simulink model "test_pkt_reorder"  (Simulink 6.2)
settings: Solver=ode45  StartTime=0.0  StopTime=200000  RelTol=1e-3
libraries: xbsIndex_r3 x556, casper_library x22, xps_library x21, simulink x1
(part 1 of 3)
settings Model: LastModifiedBy=dsp
settings DebuggingCC: SolverPrmCheckMsg=warning

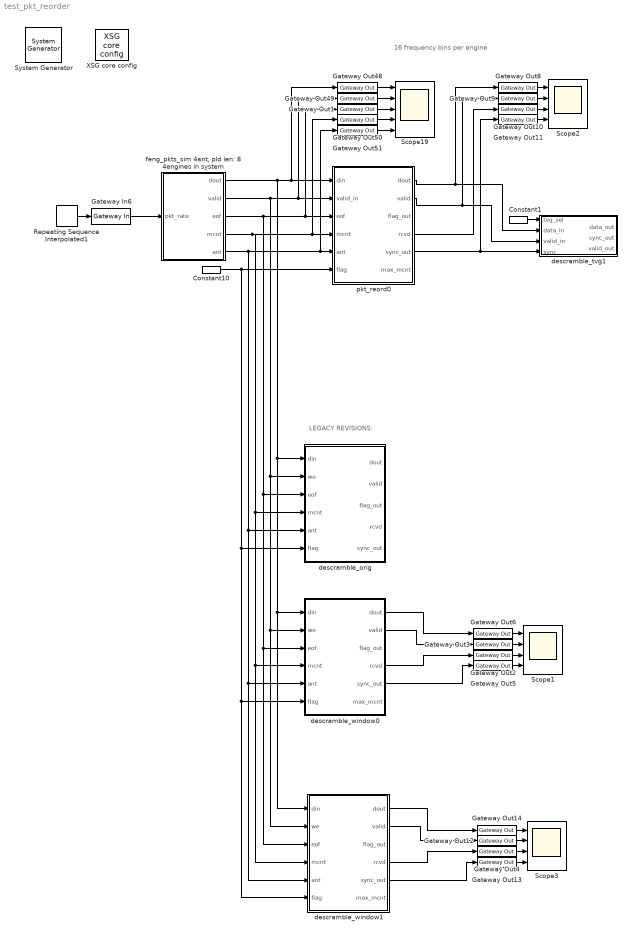
== system test_pkt_reorder ==
  note: 16 frequency bins per engine
  note: LEGACY REVISIONS:
  " System Generator" : xbsIndex_r3/ System Generator  Tag=genX  xilinxfamily=Virtex2  part=xc2v1000  speed=-4  package=bg575  synthesis_tool=XST  directory=./netlist  testbench=off  simulink_period=1  sysclk_period=100  incr_netlist=off  trim_vbits=Everywhere in SubSystem  dbl_ovrd=According to Block Masks  core_generation=According to Block Masks  run_coregen=off  deprecated_control=off  eval_field=0
      settings: AttributesFormatString=System\nGenerator
  Constant1 : xbsIndex_r3/Constant  const=0  equ=P=C  arith_type=Unsigned  n_bits=2  bin_pt=0  opselect=C  inp2=PCIN>>17  opr=+  inp1=P  carry=CIN  iostate=0  explicit_period=on  period=1  dbl_ovrd=off
  Constant10 : xbsIndex_r3/Constant  const=0  equ=P=C  arith_type=Unsigned  n_bits=1  bin_pt=0  opselect=C  inp2=PCIN>>17  opr=+  inp1=P  carry=CIN  iostate=0  explicit_period=on  period=1  dbl_ovrd=off
  Gateway In6 : xbsIndex_r3/Gateway In  arith_type=Unsigned  n_bits=1  bin_pt=0  quantization=Truncate  overflow=Wrap  period=1  timing_constraint=None  locs_specified=off  LOCs={}  needs_fixed_name=off  dbl_ovrd=off  show_param=off
      settings: xl_area=[0, 0, 0, 0, 0, 0, 0]
  Gateway Out{1..6,8..14,48..51} (17 alike) : xbsIndex_r3/Gateway Out  output_type=Double  nbits=8  bin_pt=6  arith_type=Boolean  quantization=Truncate  overflow=Wrap  hdl_port=on  timing_constraint=None  locs_specified=off  LOCs={}  needs_fixed_name=off  show_param=off
      settings: xl_area=[0, 0, 0, 0, 0, 0, 0]
  Repeating Sequence Interpolated1 : simulink/Sources/Repeating Sequence Interpolated  OutValues=[0 1].'  TimeValues=[50000 100000].'  LookUpMeth=Use Input Above  tsamp=1  OutputDataTypeScalingMode=Specify via dialog  OutDataType=float('double')  OutScaling=2^-10
  Scope1 : Scope  NumInputPorts=4
      settings: YMin=0~0~0~-1  YMax=1~1~1~1  SaveName=ScopeData5
  Scope19 : Scope  NumInputPorts=5
      settings: YMin=0~0~0~0~0  YMax=3e+014~1~1~3000~3  SaveName=ScopeData2
  Scope2 : Scope  NumInputPorts=4
      settings: YMin=0~0~0~-1  YMax=1~1~1~1
  Scope3 : Scope  NumInputPorts=4
      settings: YMin=0~0~0~-1  YMax=1~1~1~1  SaveName=ScopeData6
  XSG core config : xps_library/XSG core config  Tag=xps:xsg  hw_sys=BEE2_usr  ibob_linux=off  clk_src=sys_clk  gpio_clk_io_group=iBOB:sma  gpio_clk_bit_index=0  clk_rate=205  sample_period=1  synthesis_tool=XST  mpc_type=powerpc405
  descramble_orig : Subsystem  mask{ant_bits=2, x_int_bits=5, window_bits=3, sync_bits=11}
      mask prompts: ant_bits "Maximum Number of Antennas (2^?):"; x_int_bits "X Engine Integration Length (2^?):"; window_bits "Number of Windows to Buffer (2^?):"; sync_bits "Samples Between Sync Pulses (2^?)"
  descramble_tvg1 : Subsystem  mask{ant_bits=2, x_int_bits=5, sync_period=15}
      mask prompts: ant_bits "Number of Antennas (2^?):"; x_int_bits "X Integration Length (2^?):"; sync_period "Sync Pulse Period (2^?):"
  descramble_window0 : Subsystem  mask{ant_bits=2, xeng_bits=2, chan_bits=6, x_int_bits=5, window_bits=3}
      mask prompts: ant_bits "Maximum Number of Antennas (2^?):"; xeng_bits "Number of Xengines in the system (2^?)"; chan_bits "Number of frequency channels in the system (2^?)"; x_int_bits "X Engine Integration Length (2^?):"; window_bits "Number of Windows to Buffer (2^?):"
      mask init:
      | sync_bits=chan_bits+x_int_bits+ant_bits-xeng_bits
      | 
      | fmtstr = sprintf('Sync period: 2^%d\nPayload Len: %i', sync_bits,2^(x_int_bits - 2));
      | set_param(gcb, 'AttributesFormatString', fmtstr);
      settings: AttributesFormatString=|
      | Sync period: 2^11
      | Payload Len: 8
  descramble_window1 : Subsystem  mask{ant_bits=2, xeng_bits=2, chan_bits=6, x_int_bits=5, window_bits=3}
      mask prompts: ant_bits "Maximum Number of Antennas (2^?):"; xeng_bits "Number of Xengines in the system (2^?)"; chan_bits "Number of frequency channels in the system (2^?)"; x_int_bits "X Engine Integration Length (2^?):"; window_bits "Number of Windows to Buffer (2^?):"
      mask init:
      | sync_bits=chan_bits+x_int_bits+ant_bits-xeng_bits
      | 
      | fmtstr = sprintf('Sync period: 2^%d\nPayload Len: %i', sync_bits,2^(x_int_bits - 2));
      | set_param(gcb, 'AttributesFormatString', fmtstr);
      settings: AttributesFormatString=|
      | Sync period: 2^11
      | Payload Len: 8
  "feng_pkts_sim 4ant, pld len: 8 4engines in system" : Subsystem
  pkt_reord0 : Subsystem  mask{ant_bits=3, xeng_bits=3, chan_bits=11, x_int_bits=7, window_bits=3}
      mask prompts: ant_bits "Maximum Number of Antennas (2^?):"; xeng_bits "Number of Xengines in the system (2^?)"; chan_bits "Number of frequency channels in the system (2^?)"; x_int_bits "X Engine Integration Length (2^?):"; window_bits "Number of Windows to Buffer (2^?):"
      mask init:
      | sync_bits=chan_bits+x_int_bits+ant_bits-xeng_bits
      | 
      | fmtstr = sprintf('Sync period: 2^%d\nPayload Len: %i', sync_bits,2^(x_int_bits - 2));
      | set_param(gcb, 'AttributesFormatString', fmtstr);
      settings: AttributesFormatString=|
      | Sync period: 2^18
      | Payload Len: 32
  wires:
  Constant1/1 -> descramble_tvg1/1(tvg_sel)
  Gateway Out8/1 -> Scope2/1
  Gateway Out9/1 -> Scope2/2
  Gateway Out10/1 -> Scope2/3
  Gateway Out11/1 -> Scope2/4
  pkt_reord0/1(dout) -> Gateway Out8/1, descramble_tvg1/2(data_in)
  pkt_reord0/2(valid) -> Gateway Out9/1, descramble_tvg1/3(valid_in)
  pkt_reord0/5(sync_out) -> Gateway Out11/1, descramble_tvg1/4(sync)
  Constant10/1 -> descramble_window0/6(flag), descramble_window1/6(flag), descramble_orig/6(flag), pkt_reord0/6(flag)
  Gateway Out48/1 -> Scope19/1
  Gateway Out49/1 -> Scope19/2
  "feng_pkts_sim 4ant, pld len: 8 4engines in system"/4(mcnt) -> Gateway Out50/1, pkt_reord0/4(mcnt), descramble_window0/4(mcnt), descramble_window1/4(mcnt), descramble_orig/4(mcnt)
  "feng_pkts_sim 4ant, pld len: 8 4engines in system"/1(dout) -> Gateway Out48/1, pkt_reord0/1(din), descramble_window0/1(din), descramble_window1/1(din), descramble_orig/1(din)
  Repeating Sequence Interpolated1/1 -> Gateway In6/1
  "feng_pkts_sim 4ant, pld len: 8 4engines in system"/2(valid) -> Gateway Out49/1, pkt_reord0/2(valid_in), descramble_window0/2(we), descramble_window1/2(we), descramble_orig/2(we)
  Gateway In6/1 -> "feng_pkts_sim 4ant, pld len: 8 4engines in system"/1(pkt_rate)
  "feng_pkts_sim 4ant, pld len: 8 4engines in system"/3(eof) -> Gateway Out1/1, pkt_reord0/3(eof), descramble_window0/3(eof), descramble_window1/3(eof), descramble_orig/3(eof)
  "feng_pkts_sim 4ant, pld len: 8 4engines in system"/5(ant) -> Gateway Out51/1, pkt_reord0/5(ant), descramble_window0/5(ant), descramble_window1/5(ant), descramble_orig/5(ant)
  pkt_reord0/4(rcvd) -> Gateway Out10/1
  Gateway Out50/1 -> Scope19/4
  Gateway Out51/1 -> Scope19/5
  Gateway Out1/1 -> Scope19/3
  Gateway Out6/1 -> Scope1/1
  Gateway Out3/1 -> Scope1/2
  Gateway Out2/1 -> Scope1/3
  Gateway Out5/1 -> Scope1/4
  descramble_window0/1(dout) -> Gateway Out6/1
  descramble_window0/2(valid) -> Gateway Out3/1
  descramble_window0/4(rcvd) -> Gateway Out2/1
  descramble_window0/5(sync_out) -> Gateway Out5/1
  Gateway Out14/1 -> Scope3/1
  Gateway Out12/1 -> Scope3/2
  Gateway Out4/1 -> Scope3/3
  Gateway Out13/1 -> Scope3/4
  descramble_window1/1(dout) -> Gateway Out14/1
  descramble_window1/2(valid) -> Gateway Out12/1
  descramble_window1/4(rcvd) -> Gateway Out4/1
  descramble_window1/5(sync_out) -> Gateway Out13/1

== system test_pkt_reorder/descramble_orig ==
  note: BRAM depth is
      | X int length * # antennas * # windows
  din : Inport  Port=1  LatchInput=off
  we : Inport  Port=2  LatchInput=off
  eof : Inport  Port=3  LatchInput=off
  mcnt : Inport  Port=4  LatchInput=off
  ant : Inport  Port=5  LatchInput=off
  flag : Inport  Port=6  LatchInput=off
  Constant : xbsIndex_r3/Constant  const=0  equ=P=C  arith_type=Unsigned  n_bits=18  bin_pt=0  opselect=C  inp2=PCIN>>17  opr=+  inp1=P  carry=CIN  iostate=0  explicit_period=on  period=1  dbl_ovrd=off
  Constant1 : xbsIndex_r3/Constant  const=0  equ=P=C  arith_type=Unsigned  n_bits=1  bin_pt=0  opselect=C  inp2=PCIN>>17  opr=+  inp1=P  carry=CIN  iostate=0  explicit_period=off  period=1  dbl_ovrd=off
  Delay1 : xbsIndex_r3/Delay  latency=2  reg_retiming=off  explicit_period=off  period=1  en=off  accept_only_valid=off  init_zero=on  dbl_ovrd=off  show_param=off
      settings: xl_area=[0, 0, 0, 0, 0, 0, 0]
  Delay2 : xbsIndex_r3/Delay  latency=4  reg_retiming=off  explicit_period=off  period=1  en=off  accept_only_valid=off  init_zero=on  dbl_ovrd=off  show_param=off
      settings: xl_area=[0, 0, 0, 0, 0, 0, 0]
  Delay3 : xbsIndex_r3/Delay  latency=2  reg_retiming=off  explicit_period=off  period=1  en=off  accept_only_valid=off  init_zero=on  dbl_ovrd=off  show_param=off
      settings: xl_area=[0, 0, 0, 0, 0, 0, 0]
  Delay4 : xbsIndex_r3/Delay  latency=4  reg_retiming=off  explicit_period=off  period=1  en=off  accept_only_valid=off  init_zero=on  dbl_ovrd=off  show_param=off
      settings: xl_area=[0, 0, 0, 0, 0, 0, 0]
  Dual Port RAM : xbsIndex_r3/Dual Port RAM  depth=2^x_int_bits * 2^ant_bits * 2^window_bits  initVector=0  write_mode_A=Read Before Write  write_mode_B=Read Before Write  latency=2  mem_collision=on  init_zero=on  explicit_period=off  period=1  dbl_ovrd=off  rst_a=off  init_a=0  rst_b=off  init_b=0  show_param=off  distributed_mem=off  use_rpm=off  gen_core=off
      settings: xl_area=[0, 0, 0, 0, 0, 0, 0]
  Mux : xbsIndex_r3/Mux  inputs=2  precision=Full  arith_type="Signed  (2's comp)"  n_bits=8  bin_pt=2  quantization=Truncate  overflow=Wrap  latency=0  explicit_period=off  period=1  en=off  dbl_ovrd=off  show_param=off  mux_type=off  use_rpm=off  gen_core=off
      settings: xl_area=[0, 0, 0, 0, 0, 0, 0]
  deflagger : Subsystem
  flagger : Subsystem
  window_addr_gen : Subsystem
  dout : Outport
  valid : Outport  Port=2
  flag_out : Outport  Port=3
  rcvd : Outport  Port=4
  sync_out : Outport  Port=5
  wires:
  window_addr_gen/4(we) -> Dual Port RAM/6
  window_addr_gen/3(wr_addr) -> Dual Port RAM/4
  window_addr_gen/2(re) -> Dual Port RAM/3, Delay1/1
  window_addr_gen/1(rd_addr) -> Dual Port RAM/1
  flagger/1(dout) -> Dual Port RAM/5
  Constant/1 -> Dual Port RAM/2
  deflagger/3(rcvd) -> rcvd/1
  deflagger/2(flag) -> flag_out/1
  deflagger/1(dout) -> dout/1
  Delay1/1 -> valid/1
  we/1 -> window_addr_gen/4(valid)
  eof/1 -> window_addr_gen/3(eof)
  ant/1 -> window_addr_gen/2(ant)
  mcnt/1 -> window_addr_gen/1(mcnt)
  Delay3/1 -> sync_out/1
  window_addr_gen/5(sync_out) -> Delay3/1
  flag/1 -> Delay4/1
  Delay4/1 -> flagger/1(flag)
  din/1 -> Delay2/1
  Delay2/1 -> flagger/2(din)
  Mux/1 -> deflagger/1(din)
  Constant1/1 -> Mux/2
  Dual Port RAM/2 -> Mux/1
  Dual Port RAM/1 -> Mux/3

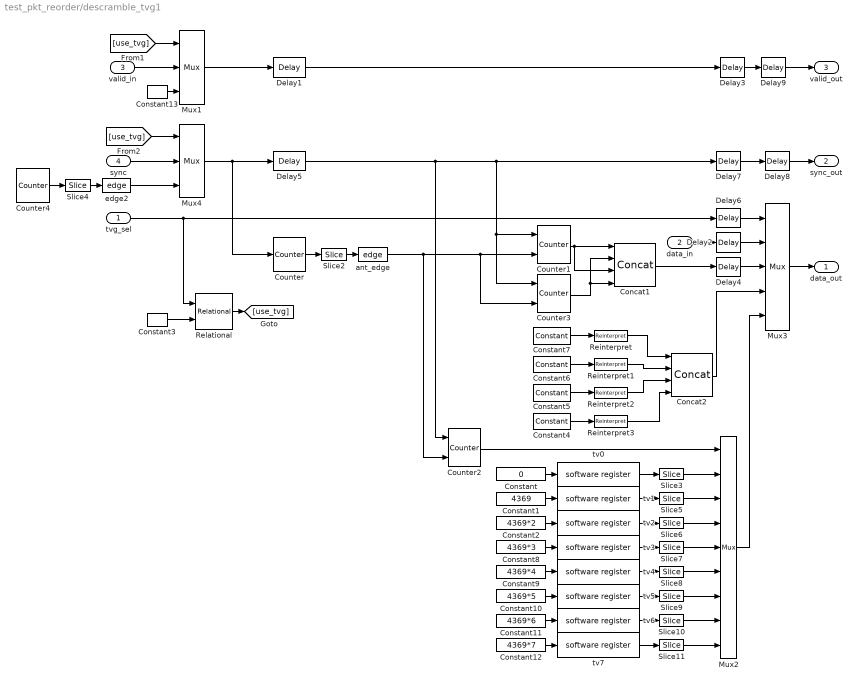
== system test_pkt_reorder/descramble_tvg1 ==
  tvg_sel : Inport  Port=1  LatchInput=off
  data_in : Inport  Port=2  LatchInput=off
  valid_in : Inport  Port=3  LatchInput=off
  sync : Inport  Port=4  LatchInput=off
  Concat1 : xbsIndex_r3/Concat  num_inputs=4  explicit_period=off  period=1  dbl_ovrd=off
  Concat2 : xbsIndex_r3/Concat  num_inputs=4  explicit_period=off  period=1  dbl_ovrd=off
  Constant : Constant  Value=0
  Constant1 : Constant  Value=4369
  Constant10 : Constant  Value=4369*5
  Constant11 : Constant  Value=4369*6
  Constant12 : Constant  Value=4369*7
  Constant13 : xbsIndex_r3/Constant  const=1  equ=P=C  arith_type=Boolean  n_bits=1  bin_pt=0  opselect=C  inp2=PCIN>>17  opr=+  inp1=P  carry=CIN  iostate=0  explicit_period=on  period=1  dbl_ovrd=off
  Constant2 : Constant  Value=4369*2
  Constant3 : xbsIndex_r3/Constant  const=0  equ=P=C  arith_type=Unsigned  n_bits=2  bin_pt=0  opselect=C  inp2=PCIN>>17  opr=+  inp1=P  carry=CIN  iostate=0  explicit_period=on  period=1  dbl_ovrd=off
  Constant4 : xbsIndex_r3/Constant  const=-0.25  equ=P=C  arith_type="Signed  (2's comp)"  n_bits=4  bin_pt=3  opselect=C  inp2=PCIN>>17  opr=+  inp1=P  carry=CIN  iostate=0  explicit_period=on  period=1  dbl_ovrd=off
  Constant5 : xbsIndex_r3/Constant  const=0.5  equ=P=C  arith_type="Signed  (2's comp)"  n_bits=4  bin_pt=3  opselect=C  inp2=PCIN>>17  opr=+  inp1=P  carry=CIN  iostate=0  explicit_period=on  period=1  dbl_ovrd=off
  Constant6 : xbsIndex_r3/Constant  const=-6/8  equ=P=C  arith_type="Signed  (2's comp)"  n_bits=4  bin_pt=3  opselect=C  inp2=PCIN>>17  opr=+  inp1=P  carry=CIN  iostate=0  explicit_period=on  period=1  dbl_ovrd=off
  Constant7 : xbsIndex_r3/Constant  const=0.1  equ=P=C  arith_type="Signed  (2's comp)"  n_bits=4  bin_pt=3  opselect=C  inp2=PCIN>>17  opr=+  inp1=P  carry=CIN  iostate=0  explicit_period=on  period=1  dbl_ovrd=off
  Constant8 : Constant  Value=4369*3
  Constant9 : Constant  Value=4369*4
  Counter : xbsIndex_r3/Counter  cnt_type=Free Running  n_bits=x_int_bits + 1  bin_pt=0  arith_type=Unsigned  start_count=0  cnt_to=Inf  cnt_by_val=1  operation=Up  explicit_period=off  period=1  load_pin=off  rst=on  en=off  dbl_ovrd=off  show_param=off  use_rpm=on  gen_core=off
      settings: xl_area=[0, 0, 0, 0, 0, 0, 0]
  Counter1 : xbsIndex_r3/Counter  cnt_type=Free Running  n_bits=4  bin_pt=0  arith_type=Unsigned  start_count=0  cnt_to=7  cnt_by_val=1  operation=Up  explicit_period=off  period=1  load_pin=off  rst=on  en=on  dbl_ovrd=off  show_param=off  use_rpm=on  gen_core=off
      settings: xl_area=[0, 0, 0, 0, 0, 0, 0]
  Counter2 : xbsIndex_r3/Counter  cnt_type=Free Running  n_bits=3  bin_pt=0  arith_type=Unsigned  start_count=0  cnt_to=7  cnt_by_val=1  operation=Up  explicit_period=off  period=1  load_pin=off  rst=on  en=on  dbl_ovrd=off  show_param=off  use_rpm=on  gen_core=off
      settings: xl_area=[0, 0, 0, 0, 0, 0, 0]
  Counter3 : xbsIndex_r3/Counter  cnt_type=Free Running  n_bits=4  bin_pt=0  arith_type=Unsigned  start_count=15  cnt_to=0  cnt_by_val=1  operation=Down  explicit_period=off  period=1  load_pin=off  rst=on  en=on  dbl_ovrd=off  show_param=off  use_rpm=on  gen_core=off
      settings: xl_area=[0, 0, 0, 0, 0, 0, 0]
  Counter4 : xbsIndex_r3/Counter  cnt_type=Free Running  n_bits=sync_period+1  bin_pt=0  arith_type=Unsigned  start_count=2^sync_period - 2  cnt_to=Inf  cnt_by_val=1  operation=Up  explicit_period=off  period=1  load_pin=off  rst=off  en=off  dbl_ovrd=off  show_param=off  use_rpm=on  gen_core=off
      settings: xl_area=[0, 0, 0, 0, 0, 0, 0]
  Delay{1,3..9} (8 alike) : xbsIndex_r3/Delay  latency=1  reg_retiming=off  explicit_period=off  period=1  en=off  accept_only_valid=off  init_zero=on  dbl_ovrd=off  show_param=off
      settings: xl_area=[0, 0, 0, 0, 0, 0, 0]
  Delay2 : xbsIndex_r3/Delay  latency=2  reg_retiming=off  explicit_period=off  period=1  en=off  accept_only_valid=off  init_zero=on  dbl_ovrd=off  show_param=off
      settings: xl_area=[0, 0, 0, 0, 0, 0, 0]
  Mux1 : xbsIndex_r3/Mux  inputs=2  precision=Full  arith_type="Signed  (2's comp)"  n_bits=8  bin_pt=2  quantization=Truncate  overflow=Wrap  latency=0  explicit_period=on  period=1  en=off  dbl_ovrd=off  show_param=off  mux_type=off  use_rpm=off  gen_core=off
      settings: xl_area=[0, 0, 0, 0, 0, 0, 0]
  Mux2 : xbsIndex_r3/Mux  inputs=8  precision=Full  arith_type="Signed  (2's comp)"  n_bits=8  bin_pt=2  quantization=Truncate  overflow=Wrap  latency=1  explicit_period=off  period=1  en=off  dbl_ovrd=off  show_param=off  mux_type=off  use_rpm=off  gen_core=off
      settings: xl_area=[0, 0, 0, 0, 0, 0, 0]
  Mux3 : xbsIndex_r3/Mux  inputs=4  precision=Full  arith_type="Signed  (2's comp)"  n_bits=8  bin_pt=2  quantization=Truncate  overflow=Wrap  latency=1  explicit_period=off  period=1  en=off  dbl_ovrd=off  show_param=off  mux_type=off  use_rpm=off  gen_core=off
      settings: xl_area=[0, 0, 0, 0, 0, 0, 0]
  Mux4 : xbsIndex_r3/Mux  inputs=2  precision=Full  arith_type="Signed  (2's comp)"  n_bits=8  bin_pt=2  quantization=Truncate  overflow=Wrap  latency=0  explicit_period=on  period=1  en=off  dbl_ovrd=off  show_param=off  mux_type=off  use_rpm=off  gen_core=off
      settings: xl_area=[0, 0, 0, 0, 0, 0, 0]
  Reinterpret{,1..3} (4 alike) : xbsIndex_r3/Reinterpret  force_arith_type=on  arith_type=Unsigned  force_bin_pt=on  bin_pt=0  force_valid=on
  Relational : xbsIndex_r3/Relational  mode=a!=b  latency=1  explicit_period=off  period=1  en=off  dbl_ovrd=off  show_param=off
      settings: xl_area=[0, 0, 0, 0, 0, 0, 0]
  Slice{3,5..11} (8 alike) : xbsIndex_r3/Slice  mode=Lower Bit Location + Width  nbits=16  bit1=0  base1=MSB of Input  bit0=0  base0=LSB of Input  boolean_output=off  explicit_period=off  period=1  dbl_ovrd=off
  Slice2 : xbsIndex_r3/Slice  mode=Lower Bit Location + Width  nbits=1  bit1=0  base1=MSB of Input  bit0=x_int_bits  base0=LSB of Input  boolean_output=on  explicit_period=off  period=1  dbl_ovrd=off
  Slice4 : xbsIndex_r3/Slice  mode=Lower Bit Location + Width  nbits=1  bit1=0  base1=MSB of Input  bit0=sync_period  base0=LSB of Input  boolean_output=on  explicit_period=off  period=1  dbl_ovrd=off
  ant_edge : casper_library/Misc/edge
  edge2 : casper_library/Misc/edge
  tv0 : xps_library/software register  Tag=xps:sw_reg  io_dir=From Processor  arith_type=Unsigned  bitwidth=32  bin_pt=0  sample_period=1  gw_name=test_pkt_reorder_descramble_tvg1_tv0_user_data_out
  tv1 : xps_library/software register  Tag=xps:sw_reg  io_dir=From Processor  arith_type=Unsigned  bitwidth=32  bin_pt=0  sample_period=1  gw_name=test_pkt_reorder_descramble_tvg1_tv1_user_data_out
  tv2 : xps_library/software register  Tag=xps:sw_reg  io_dir=From Processor  arith_type=Unsigned  bitwidth=32  bin_pt=0  sample_period=1  gw_name=test_pkt_reorder_descramble_tvg1_tv2_user_data_out
  tv3 : xps_library/software register  Tag=xps:sw_reg  io_dir=From Processor  arith_type=Unsigned  bitwidth=32  bin_pt=0  sample_period=1  gw_name=test_pkt_reorder_descramble_tvg1_tv3_user_data_out
  tv4 : xps_library/software register  Tag=xps:sw_reg  io_dir=From Processor  arith_type=Unsigned  bitwidth=32  bin_pt=0  sample_period=1  gw_name=test_pkt_reorder_descramble_tvg1_tv4_user_data_out
  tv5 : xps_library/software register  Tag=xps:sw_reg  io_dir=From Processor  arith_type=Unsigned  bitwidth=32  bin_pt=0  sample_period=1  gw_name=test_pkt_reorder_descramble_tvg1_tv5_user_data_out
  tv6 : xps_library/software register  Tag=xps:sw_reg  io_dir=From Processor  arith_type=Unsigned  bitwidth=32  bin_pt=0  sample_period=1  gw_name=test_pkt_reorder_descramble_tvg1_tv6_user_data_out
  tv7 : xps_library/software register  Tag=xps:sw_reg  io_dir=From Processor  arith_type=Unsigned  bitwidth=32  bin_pt=0  sample_period=1  gw_name=test_pkt_reorder_descramble_tvg1_tv7_user_data_out
  data_out : Outport
  sync_out : Outport  Port=2
  valid_out : Outport  Port=3
  wires:
  Counter1/1 -> Concat1/1, Concat1/3
  ant_edge/1 -> Counter2/2, Counter1/2, Counter3/2
  Counter/1 -> Slice2/1
  Slice2/1 -> ant_edge/1
  Concat1/1 -> Delay4/1
  Delay8/1 -> sync_out/1
  data_in/1 -> Delay2/1
  Delay2/1 -> Mux3/2
  Mux3/1 -> data_out/1
  Delay3/1 -> Delay9/1
  tvg_sel/1 -> Delay6/1, Relational/1
  Delay6/1 -> Mux3/1
  Constant3/1 -> Relational/2
  Concat2/1 -> Mux3/4
  Counter3/1 -> Concat1/2, Concat1/4
  Delay7/1 -> Delay8/1
  Delay5/1 -> Delay7/1, Counter1/1, Counter3/1, Counter2/1
  Delay4/1 -> Mux3/3
  Relational/1 -> [use_tvg]
  [use_tvg] -> Mux4/1
  Slice4/1 -> edge2/1
  Counter4/1 -> Slice4/1
  sync/1 -> Mux4/2
  Mux4/1 -> Delay5/1, Counter/1
  tv0/1 -> Slice3/1
  Constant/1 -> tv0/1
  Mux2/1 -> Mux3/5
  Slice3/1 -> Mux2/2
  Counter2/1 -> Mux2/1
  tv1/1 -> Slice5/1
  tv2/1 -> Slice6/1
  tv3/1 -> Slice7/1
  tv4/1 -> Slice8/1
  tv5/1 -> Slice9/1
  tv6/1 -> Slice10/1
  tv7/1 -> Slice11/1
  Slice5/1 -> Mux2/3
  Slice6/1 -> Mux2/4
  Slice7/1 -> Mux2/5
  Slice8/1 -> Mux2/6
  Slice9/1 -> Mux2/7
  Slice10/1 -> Mux2/8
  Slice11/1 -> Mux2/9
  edge2/1 -> Mux4/3
  Constant7/1 -> Reinterpret/1
  Constant6/1 -> Reinterpret1/1
  Constant5/1 -> Reinterpret2/1
  Constant4/1 -> Reinterpret3/1
  Reinterpret/1 -> Concat2/1
  Reinterpret1/1 -> Concat2/2
  Reinterpret2/1 -> Concat2/3
  Reinterpret3/1 -> Concat2/4
  Constant1/1 -> tv1/1
  Constant2/1 -> tv2/1
  Constant12/1 -> tv7/1
  Constant11/1 -> tv6/1
  Constant10/1 -> tv5/1
  Constant9/1 -> tv4/1
  Constant8/1 -> tv3/1
  Delay9/1 -> valid_out/1
  valid_in/1 -> Mux1/2
  Mux1/1 -> Delay1/1
  [use_tvg] -> Mux1/1
  Constant13/1 -> Mux1/3
  Delay1/1 -> Delay3/1

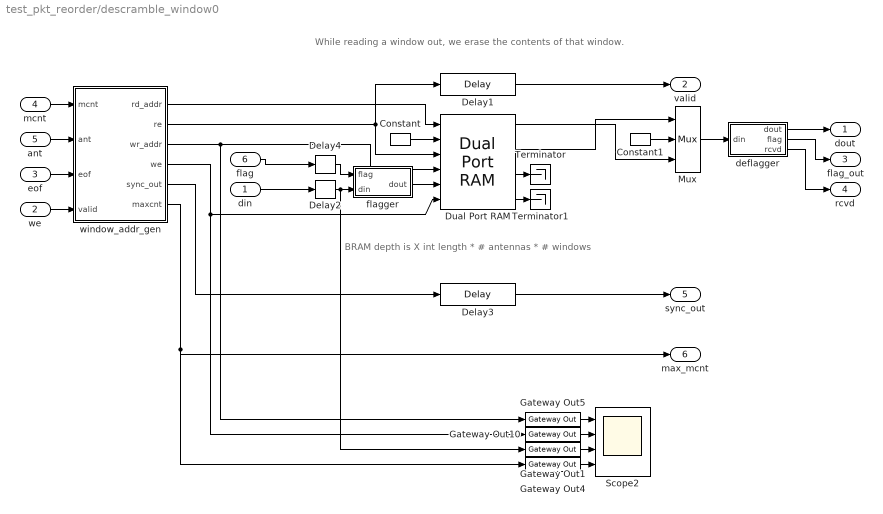
== system test_pkt_reorder/descramble_window0 ==
  note: BRAM depth is
      | X int length * # antennas * # windows
  note: While reading a window out,
      | we erase the contents of that window.
  din : Inport  Port=1  LatchInput=off
  we : Inport  Port=2  LatchInput=off
  eof : Inport  Port=3  LatchInput=off
  mcnt : Inport  Port=4  LatchInput=off
  ant : Inport  Port=5  LatchInput=off
  flag : Inport  Port=6  LatchInput=off
  Constant : xbsIndex_r3/Constant  const=0  equ=P=C  arith_type=Unsigned  n_bits=18  bin_pt=0  opselect=C  inp2=PCIN>>17  opr=+  inp1=P  carry=CIN  iostate=0  explicit_period=on  period=1  dbl_ovrd=off
  Constant1 : xbsIndex_r3/Constant  const=0  equ=P=C  arith_type=Unsigned  n_bits=1  bin_pt=0  opselect=C  inp2=PCIN>>17  opr=+  inp1=P  carry=CIN  iostate=0  explicit_period=off  period=1  dbl_ovrd=off
  Delay1 : xbsIndex_r3/Delay  latency=2  reg_retiming=on  explicit_period=off  period=1  en=off  accept_only_valid=off  init_zero=on  dbl_ovrd=off  show_param=off
      settings: xl_area=[0, 0, 0, 0, 0, 0, 0]
  Delay2 : xbsIndex_r3/Delay  latency=4  reg_retiming=off  explicit_period=off  period=1  en=off  accept_only_valid=off  init_zero=on  dbl_ovrd=off  show_param=off
      settings: xl_area=[0, 0, 0, 0, 0, 0, 0]
  Delay3 : xbsIndex_r3/Delay  latency=2  reg_retiming=on  explicit_period=off  period=1  en=off  accept_only_valid=off  init_zero=on  dbl_ovrd=off  show_param=off
      settings: xl_area=[0, 0, 0, 0, 0, 0, 0]
  Delay4 : xbsIndex_r3/Delay  latency=4  reg_retiming=off  explicit_period=off  period=1  en=off  accept_only_valid=off  init_zero=on  dbl_ovrd=off  show_param=off
      settings: xl_area=[0, 0, 0, 0, 0, 0, 0]
  Dual Port RAM : xbsIndex_r3/Dual Port RAM  depth=2^x_int_bits * 2^ant_bits * 2^window_bits  initVector=1  write_mode_A=Read Before Write  write_mode_B=Read Before Write  latency=2  mem_collision=on  init_zero=on  explicit_period=on  period=1  dbl_ovrd=off  rst_a=off  init_a=0  rst_b=off  init_b=0  show_param=off  distributed_mem=off  use_rpm=off  gen_core=off
      settings: xl_area=[0, 0, 0, 0, 0, 0, 0]
  Gateway Out{1,4..5,10} (4 alike) : xbsIndex_r3/Gateway Out  output_type=Double  nbits=8  bin_pt=6  arith_type=Boolean  quantization=Truncate  overflow=Wrap  hdl_port=on  timing_constraint=None  locs_specified=off  LOCs={}  needs_fixed_name=off  show_param=off
      settings: xl_area=[0, 0, 0, 0, 0, 0, 0]
  Mux : xbsIndex_r3/Mux  inputs=2  precision=Full  arith_type="Signed  (2's comp)"  n_bits=8  bin_pt=2  quantization=Truncate  overflow=Wrap  latency=0  explicit_period=off  period=1  en=off  dbl_ovrd=off  show_param=off  mux_type=off  use_rpm=off  gen_core=off
      settings: xl_area=[0, 0, 0, 0, 0, 0, 0]
  Scope2 : Scope  NumInputPorts=4
      settings: YMin=0~0~0~-1  YMax=1~1~1~1
  Terminator : Terminator
  Terminator1 : Terminator
  deflagger : Subsystem
  flagger : Subsystem
  window_addr_gen : Subsystem
  dout : Outport
  valid : Outport  Port=2
  flag_out : Outport  Port=3
  rcvd : Outport  Port=4
  sync_out : Outport  Port=5
  max_mcnt : Outport  Port=6
  wires:
  window_addr_gen/4(we) -> Dual Port RAM/6, Gateway Out10/1
  window_addr_gen/3(wr_addr) -> Dual Port RAM/4, Gateway Out5/1
  window_addr_gen/2(re) -> Delay1/1, Dual Port RAM/3
  window_addr_gen/1(rd_addr) -> Dual Port RAM/1
  flagger/1(dout) -> Dual Port RAM/5
  Constant/1 -> Dual Port RAM/2
  deflagger/3(rcvd) -> rcvd/1
  deflagger/2(flag) -> flag_out/1
  deflagger/1(dout) -> dout/1
  Delay1/1 -> valid/1
  we/1 -> window_addr_gen/4(valid)
  eof/1 -> window_addr_gen/3(eof)
  ant/1 -> window_addr_gen/2(ant)
  mcnt/1 -> window_addr_gen/1(mcnt)
  window_addr_gen/5(sync_out) -> Delay3/1
  flag/1 -> Delay4/1
  Delay4/1 -> flagger/1(flag)
  din/1 -> Delay2/1
  Delay2/1 -> flagger/2(din), Gateway Out1/1
  window_addr_gen/6(maxcnt) -> max_mcnt/1, Gateway Out4/1
  Delay3/1 -> sync_out/1
  Dual Port RAM/3 -> Terminator/1
  Dual Port RAM/4 -> Terminator1/1
  Constant1/1 -> Mux/2
  Dual Port RAM/2 -> Mux/1
  Dual Port RAM/1 -> Mux/3
  Mux/1 -> deflagger/1(din)
  Gateway Out5/1 -> Scope2/1
  Gateway Out10/1 -> Scope2/2
  Gateway Out1/1 -> Scope2/3
  Gateway Out4/1 -> Scope2/4

== system test_pkt_reorder/descramble_window1 ==
  note: BRAM depth is
      | X int length * # antennas * # windows
  note: While reading a window out,
      | we erase the contents of that window.
  din : Inport  Port=1  LatchInput=off
  we : Inport  Port=2  LatchInput=off
  eof : Inport  Port=3  LatchInput=off
  mcnt : Inport  Port=4  LatchInput=off
  ant : Inport  Port=5  LatchInput=off
  flag : Inport  Port=6  LatchInput=off
  Constant : xbsIndex_r3/Constant  const=0  equ=P=C  arith_type=Unsigned  n_bits=18  bin_pt=0  opselect=C  inp2=PCIN>>17  opr=+  inp1=P  carry=CIN  iostate=0  explicit_period=on  period=1  dbl_ovrd=off
  Constant1 : xbsIndex_r3/Constant  const=0  equ=P=C  arith_type=Unsigned  n_bits=1  bin_pt=0  opselect=C  inp2=PCIN>>17  opr=+  inp1=P  carry=CIN  iostate=0  explicit_period=off  period=1  dbl_ovrd=off
  Delay1 : xbsIndex_r3/Delay  latency=2  reg_retiming=on  explicit_period=off  period=1  en=off  accept_only_valid=off  init_zero=on  dbl_ovrd=off  show_param=off
      settings: xl_area=[0, 0, 0, 0, 0, 0, 0]
  Delay2 : xbsIndex_r3/Delay  latency=4  reg_retiming=off  explicit_period=off  period=1  en=off  accept_only_valid=off  init_zero=on  dbl_ovrd=off  show_param=off
      settings: xl_area=[0, 0, 0, 0, 0, 0, 0]
  Delay3 : xbsIndex_r3/Delay  latency=2  reg_retiming=on  explicit_period=off  period=1  en=off  accept_only_valid=off  init_zero=on  dbl_ovrd=off  show_param=off
      settings: xl_area=[0, 0, 0, 0, 0, 0, 0]
  Delay4 : xbsIndex_r3/Delay  latency=4  reg_retiming=off  explicit_period=off  period=1  en=off  accept_only_valid=off  init_zero=on  dbl_ovrd=off  show_param=off
      settings: xl_area=[0, 0, 0, 0, 0, 0, 0]
  Dual Port RAM : xbsIndex_r3/Dual Port RAM  depth=2^x_int_bits * 2^ant_bits * 2^window_bits  initVector=1  write_mode_A=Read Before Write  write_mode_B=Read Before Write  latency=2  mem_collision=on  init_zero=on  explicit_period=on  period=1  dbl_ovrd=off  rst_a=off  init_a=0  rst_b=off  init_b=0  show_param=off  distributed_mem=off  use_rpm=off  gen_core=off
      settings: xl_area=[0, 0, 0, 0, 0, 0, 0]
  Gateway Out{1,4..5,10} (4 alike) : xbsIndex_r3/Gateway Out  output_type=Double  nbits=8  bin_pt=6  arith_type=Boolean  quantization=Truncate  overflow=Wrap  hdl_port=on  timing_constraint=None  locs_specified=off  LOCs={}  needs_fixed_name=off  show_param=off
      settings: xl_area=[0, 0, 0, 0, 0, 0, 0]
  Mux : xbsIndex_r3/Mux  inputs=2  precision=Full  arith_type="Signed  (2's comp)"  n_bits=8  bin_pt=2  quantization=Truncate  overflow=Wrap  latency=0  explicit_period=off  period=1  en=off  dbl_ovrd=off  show_param=off  mux_type=off  use_rpm=off  gen_core=off
      settings: xl_area=[0, 0, 0, 0, 0, 0, 0]
  Scope2 : Scope  NumInputPorts=4
      settings: YMin=0~0~0~-1  YMax=1~1~1~1
  Terminator : Terminator
  Terminator1 : Terminator
  deflagger : Subsystem
  flagger : Subsystem
  window_addr_gen : Subsystem
  dout : Outport
  valid : Outport  Port=2
  flag_out : Outport  Port=3
  rcvd : Outport  Port=4
  sync_out : Outport  Port=5
  max_mcnt : Outport  Port=6
  wires:
  window_addr_gen/4(we) -> Dual Port RAM/6, Gateway Out10/1
  window_addr_gen/3(wr_addr) -> Dual Port RAM/4, Gateway Out5/1
  window_addr_gen/2(re) -> Delay1/1, Dual Port RAM/3
  window_addr_gen/1(rd_addr) -> Dual Port RAM/1
  flagger/1(dout) -> Dual Port RAM/5
  Constant/1 -> Dual Port RAM/2
  deflagger/3(rcvd) -> rcvd/1
  deflagger/2(flag) -> flag_out/1
  deflagger/1(dout) -> dout/1
  Delay1/1 -> valid/1
  we/1 -> window_addr_gen/4(valid)
  eof/1 -> window_addr_gen/3(eof)
  ant/1 -> window_addr_gen/2(ant)
  mcnt/1 -> window_addr_gen/1(mcnt)
  window_addr_gen/5(sync_out) -> Delay3/1
  flag/1 -> Delay4/1
  Delay4/1 -> flagger/1(flag)
  din/1 -> Delay2/1
  Delay2/1 -> flagger/2(din), Gateway Out1/1
  window_addr_gen/6(maxcnt) -> max_mcnt/1, Gateway Out4/1
  Delay3/1 -> sync_out/1
  Dual Port RAM/3 -> Terminator/1
  Dual Port RAM/4 -> Terminator1/1
  Constant1/1 -> Mux/2
  Dual Port RAM/2 -> Mux/1
  Dual Port RAM/1 -> Mux/3
  Mux/1 -> deflagger/1(din)
  Gateway Out5/1 -> Scope2/1
  Gateway Out10/1 -> Scope2/2
  Gateway Out1/1 -> Scope2/3
  Gateway Out4/1 -> Scope2/4

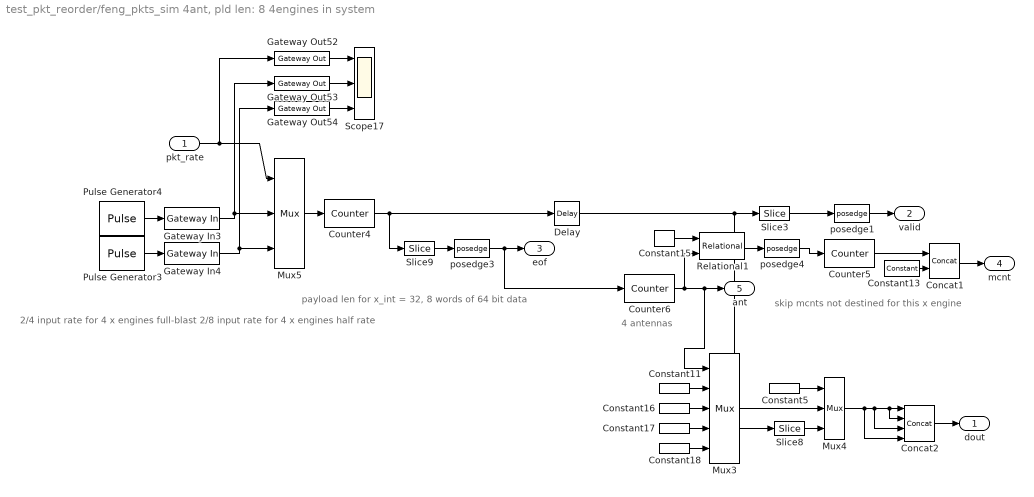
== system test_pkt_reorder/feng_pkts_sim 4ant, pld len: 8 4engines in system ==
  note: 2/4 input rate for 4 x engines full-blast
      | 2/8 input rate for 4 x engines half rate
  note: 4 antennas
  note: skip mcnts not destined
      | for this x engine
  note: payload len
      | for x_int = 32,
      | 8 words of 64 bit data
  pkt_rate : Inport  Port=1  LatchInput=off
  Concat1 : xbsIndex_r3/Concat  num_inputs=2  explicit_period=off  period=1  dbl_ovrd=off
  Concat2 : xbsIndex_r3/Concat  num_inputs=4  explicit_period=off  period=1  dbl_ovrd=off
  Constant11 : xbsIndex_r3/Constant  const=1  equ=P=C  arith_type=Unsigned  n_bits=16  bin_pt=0  opselect=C  inp2=PCIN>>17  opr=+  inp1=P  carry=CIN  iostate=0  explicit_period=on  period=1  dbl_ovrd=off
  Constant13 : xbsIndex_r3/Constant  const=0  equ=P=C  arith_type=Unsigned  n_bits=2  bin_pt=0  opselect=C  inp2=PCIN>>17  opr=+  inp1=P  carry=CIN  iostate=0  explicit_period=on  period=1  dbl_ovrd=off
  Constant15 : xbsIndex_r3/Constant  const=0  equ=P=C  arith_type=Unsigned  n_bits=3  bin_pt=0  opselect=C  inp2=PCIN>>17  opr=+  inp1=P  carry=CIN  iostate=0  explicit_period=on  period=1  dbl_ovrd=off
  Constant16 : xbsIndex_r3/Constant  const=0  equ=P=C  arith_type=Unsigned  n_bits=16  bin_pt=0  opselect=C  inp2=PCIN>>17  opr=+  inp1=P  carry=CIN  iostate=0  explicit_period=on  period=1  dbl_ovrd=off
  Constant17 : xbsIndex_r3/Constant  const=0  equ=P=C  arith_type=Unsigned  n_bits=16  bin_pt=0  opselect=C  inp2=PCIN>>17  opr=+  inp1=P  carry=CIN  iostate=0  explicit_period=on  period=1  dbl_ovrd=off
  Constant18 : xbsIndex_r3/Constant  const=0  equ=P=C  arith_type=Unsigned  n_bits=16  bin_pt=0  opselect=C  inp2=PCIN>>17  opr=+  inp1=P  carry=CIN  iostate=0  explicit_period=on  period=1  dbl_ovrd=off
  Constant5 : xbsIndex_r3/Constant  const=0  equ=P=C  arith_type=Unsigned  n_bits=1  bin_pt=0  opselect=C  inp2=PCIN>>17  opr=+  inp1=P  carry=CIN  iostate=0  explicit_period=on  period=1  dbl_ovrd=off
  Counter4 : xbsIndex_r3/Counter  cnt_type=Free Running  n_bits=32  bin_pt=0  arith_type=Unsigned  start_count=0  cnt_to=32  cnt_by_val=1  operation=Up  explicit_period=off  period=1  load_pin=off  rst=off  en=on  dbl_ovrd=off  show_param=off  use_rpm=on  gen_core=off
      settings: xl_area=[0, 0, 0, 0, 0, 0, 0]
  Counter5 : xbsIndex_r3/Counter  cnt_type=Free Running  n_bits=48-2  bin_pt=0  arith_type=Unsigned  start_count=0  cnt_to=Inf  cnt_by_val=1  operation=Up  explicit_period=off  period=1  load_pin=off  rst=off  en=on  dbl_ovrd=off  show_param=off  use_rpm=on  gen_core=off
      settings: xl_area=[0, 0, 0, 0, 0, 0, 0]
  Counter6 : xbsIndex_r3/Counter  cnt_type=Free Running  n_bits=2  bin_pt=0  arith_type=Unsigned  start_count=0  cnt_to=Inf  cnt_by_val=1  operation=Up  explicit_period=off  period=1  load_pin=off  rst=off  en=on  dbl_ovrd=off  show_param=off  use_rpm=on  gen_core=off
      settings: xl_area=[0, 0, 0, 0, 0, 0, 0]
  Delay : xbsIndex_r3/Delay  latency=1  reg_retiming=off  explicit_period=off  period=1  en=off  accept_only_valid=off  init_zero=on  dbl_ovrd=off  show_param=off
      settings: xl_area=[0, 0, 0, 0, 0, 0, 0]
  Gateway In3 : xbsIndex_r3/Gateway In  arith_type=Boolean  n_bits=8  bin_pt=6  quantization=Truncate  overflow=Wrap  period=1  timing_constraint=None  locs_specified=off  LOCs={}  needs_fixed_name=off  dbl_ovrd=off  show_param=off
      settings: xl_area=[0, 0, 0, 0, 0, 0, 0]
  Gateway In4 : xbsIndex_r3/Gateway In  arith_type=Boolean  n_bits=8  bin_pt=6  quantization=Truncate  overflow=Wrap  period=1  timing_constraint=None  locs_specified=off  LOCs={}  needs_fixed_name=off  dbl_ovrd=off  show_param=off
      settings: xl_area=[0, 0, 0, 0, 0, 0, 0]
  Gateway Out52 : xbsIndex_r3/Gateway Out  output_type=Double  nbits=8  bin_pt=6  arith_type=Boolean  quantization=Truncate  overflow=Wrap  hdl_port=on  timing_constraint=None  locs_specified=off  LOCs={}  needs_fixed_name=off  show_param=off
      settings: xl_area=[0, 0, 0, 0, 0, 0, 0]
  Gateway Out53 : xbsIndex_r3/Gateway Out  output_type=Double  nbits=8  bin_pt=6  arith_type=Boolean  quantization=Truncate  overflow=Wrap  hdl_port=on  timing_constraint=None  locs_specified=off  LOCs={}  needs_fixed_name=off  show_param=off
      settings: xl_area=[0, 0, 0, 0, 0, 0, 0]
  Gateway Out54 : xbsIndex_r3/Gateway Out  output_type=Double  nbits=8  bin_pt=6  arith_type=Boolean  quantization=Truncate  overflow=Wrap  hdl_port=on  timing_constraint=None  locs_specified=off  LOCs={}  needs_fixed_name=off  show_param=off
      settings: xl_area=[0, 0, 0, 0, 0, 0, 0]
  Mux3 : xbsIndex_r3/Mux  inputs=4  precision=Full  arith_type="Signed  (2's comp)"  n_bits=8  bin_pt=2  quantization=Truncate  overflow=Wrap  latency=0  explicit_period=off  period=1  en=off  dbl_ovrd=off  show_param=off  mux_type=off  use_rpm=off  gen_core=off
      settings: xl_area=[0, 0, 0, 0, 0, 0, 0]
  Mux4 : xbsIndex_r3/Mux  inputs=2  precision=Full  arith_type="Signed  (2's comp)"  n_bits=8  bin_pt=2  quantization=Truncate  overflow=Wrap  latency=0  explicit_period=off  period=1  en=off  dbl_ovrd=off  show_param=off  mux_type=off  use_rpm=off  gen_core=off
      settings: xl_area=[0, 0, 0, 0, 0, 0, 0]
  Mux5 : xbsIndex_r3/Mux  inputs=2  precision=Full  arith_type="Signed  (2's comp)"  n_bits=8  bin_pt=2  quantization=Truncate  overflow=Wrap  latency=0  explicit_period=off  period=1  en=off  dbl_ovrd=off  show_param=off  mux_type=off  use_rpm=off  gen_core=off
      settings: xl_area=[0, 0, 0, 0, 0, 0, 0]
  Pulse Generator3 : DiscretePulseGenerator  Period=4  PulseWidth=2
  Pulse Generator4 : DiscretePulseGenerator  PulseWidth=2
  Relational1 : xbsIndex_r3/Relational  mode=a=b  latency=1  explicit_period=off  period=1  en=off  dbl_ovrd=off  show_param=off
      settings: xl_area=[0, 0, 0, 0, 0, 0, 0]
  Scope17 : Scope  NumInputPorts=3
      settings: YMin=-1~0~0  YMax=1~1~1
  Slice3 : xbsIndex_r3/Slice  mode=Lower Bit Location + Width  nbits=1  bit1=0  base1=MSB of Input  bit0=0  base0=LSB of Input  boolean_output=on  explicit_period=off  period=1  dbl_ovrd=off
  Slice8 : xbsIndex_r3/Slice  mode=Lower Bit Location + Width  nbits=16  bit1=0  base1=MSB of Input  bit0=1  base0=LSB of Input  boolean_output=on  explicit_period=off  period=1  dbl_ovrd=off
  Slice9 : xbsIndex_r3/Slice  mode=Lower Bit Location + Width  nbits=1  bit1=0  base1=MSB of Input  bit0=4  base0=LSB of Input  boolean_output=on  explicit_period=off  period=1  dbl_ovrd=off
  posedge1 : casper_library/Misc/posedge  Tag=Rising Edge Detector
  posedge3 : casper_library/Misc/posedge  Tag=Rising Edge Detector
  posedge4 : casper_library/Misc/posedge  Tag=Rising Edge Detector
  dout : Outport
  valid : Outport  Port=2
  eof : Outport  Port=3
  mcnt : Outport  Port=4
  ant : Outport  Port=5
  wires:
  Constant13/1 -> Concat1/2
  Counter5/1 -> Concat1/1
  Counter6/1 -> Relational1/2, Mux3/1, ant/1
  Relational1/1 -> posedge4/1
  Constant15/1 -> Relational1/1
  Slice3/1 -> posedge1/1
  Counter4/1 -> Slice9/1, Delay/1
  Mux4/1 -> Concat2/4, Concat2/3, Concat2/1, Concat2/2
  Slice9/1 -> posedge3/1
  posedge3/1 -> eof/1, Counter6/1
  posedge4/1 -> Counter5/1
  Pulse Generator3/1 -> Gateway In4/1
  Constant11/1 -> Mux3/2
  Constant16/1 -> Mux3/3
  Constant17/1 -> Mux3/4
  Constant18/1 -> Mux3/5
  Mux3/1 -> Mux4/2
  Slice8/1 -> Mux4/3
  Constant5/1 -> Mux4/1
  Pulse Generator4/1 -> Gateway In3/1
  Mux5/1 -> Counter4/1
  Gateway In3/1 -> Gateway Out53/1, Mux5/2
  Gateway In4/1 -> Gateway Out54/1, Mux5/3
  pkt_rate/1 -> Gateway Out52/1, Mux5/1
  Gateway Out52/1 -> Scope17/1
  Gateway Out53/1 -> Scope17/2
  Gateway Out54/1 -> Scope17/3
  Concat2/1 -> dout/1
  posedge1/1 -> valid/1
  Concat1/1 -> mcnt/1
  Delay/1 -> Slice3/1, Slice8/1

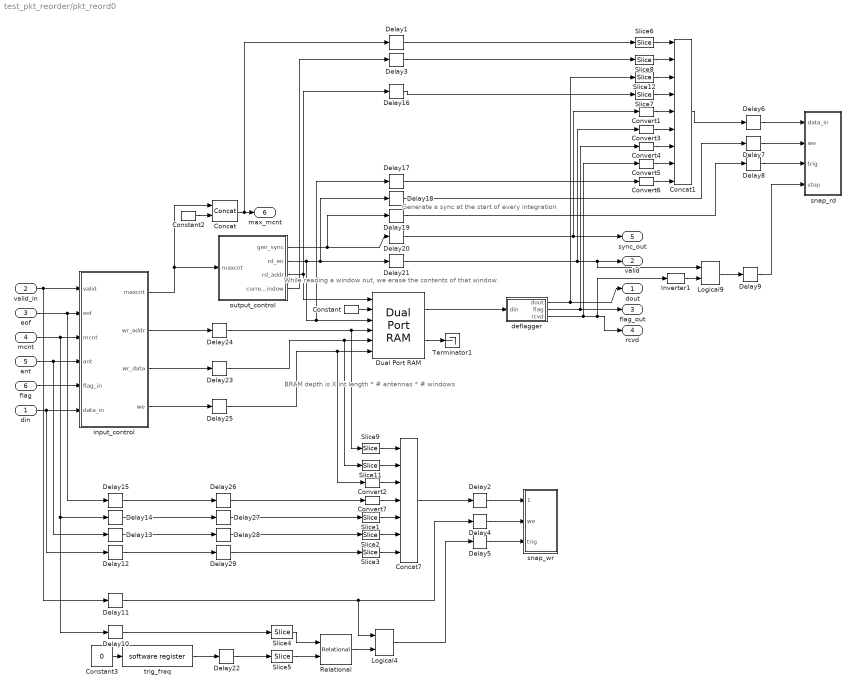
== system test_pkt_reorder/pkt_reord0 ==
  note: BRAM depth is
      | X int length * # antennas * # windows
  note: While reading a window out,
      | we erase the contents of that window.
  note: Generate a sync at the
      | start of every integration
  din : Inport  Port=1  LatchInput=off
  valid_in : Inport  Port=2  LatchInput=off
  eof : Inport  Port=3  LatchInput=off
  mcnt : Inport  Port=4  LatchInput=off
  ant : Inport  Port=5  LatchInput=off
  flag : Inport  Port=6  LatchInput=off
  Concat : xbsIndex_r3/Concat  num_inputs=2  explicit_period=off  period=1  dbl_ovrd=off
  Concat1 : xbsIndex_r3/Concat  num_inputs=9  explicit_period=off  period=1  dbl_ovrd=off
  Concat7 : xbsIndex_r3/Concat  num_inputs=7  explicit_period=off  period=1  dbl_ovrd=off
  Constant : xbsIndex_r3/Constant  const=0  equ=P=C  arith_type=Unsigned  n_bits=18  bin_pt=0  opselect=C  inp2=PCIN>>17  opr=+  inp1=P  carry=CIN  iostate=0  explicit_period=on  period=1  dbl_ovrd=off
  Constant2 : xbsIndex_r3/Constant  const=2^(xeng_bits)-1  equ=P=C  arith_type=Unsigned  n_bits=xeng_bits  bin_pt=0  opselect=C  inp2=PCIN>>17  opr=+  inp1=P  carry=CIN  iostate=0  explicit_period=on  period=1  dbl_ovrd=off
  Constant3 : Constant  Value=0
  Convert{1..7} (7 alike) : xbsIndex_r3/Convert  arith_type=Unsigned  n_bits=1  bin_pt=0  quantization=Truncate  overflow=Wrap  latency=0  explicit_period=off  period=1  dbl_ovrd=off  show_param=off  inserted_by_tool=off  pipeline=off
      settings: xl_area=[0, 0, 0, 0, 0, 0, 0]
  Delay{1,3,10,16..22} (10 alike) : xbsIndex_r3/Delay  latency=3  reg_retiming=on  explicit_period=on  period=1  en=off  accept_only_valid=off  init_zero=on  dbl_ovrd=off  show_param=off
      settings: xl_area=[0, 0, 0, 0, 0, 0, 0]
  Delay{11..15} (5 alike) : xbsIndex_r3/Delay  latency=4  reg_retiming=on  explicit_period=on  period=1  en=off  accept_only_valid=off  init_zero=on  dbl_ovrd=off  show_param=off
      settings: xl_area=[0, 0, 0, 0, 0, 0, 0]
  Delay{2,4..9,23..29} (14 alike) : xbsIndex_r3/Delay  latency=2  reg_retiming=on  explicit_period=on  period=1  en=off  accept_only_valid=off  init_zero=on  dbl_ovrd=off  show_param=off
      settings: xl_area=[0, 0, 0, 0, 0, 0, 0]
  Dual Port RAM : xbsIndex_r3/Dual Port RAM  depth=2^x_int_bits * 2^ant_bits * 2^window_bits  initVector=1  write_mode_A=Read Before Write  write_mode_B=Read Before Write  latency=3  mem_collision=off  init_zero=on  explicit_period=on  period=1  dbl_ovrd=off  rst_a=off  init_a=0  rst_b=off  init_b=0  show_param=off  distributed_mem=off  use_rpm=off  gen_core=off
      settings: xl_area=[0, 0, 0, 0, 0, 0, 0]
  Inverter1 : xbsIndex_r3/Inverter  latency=0  explicit_period=off  period=1  en=off  dbl_ovrd=off  show_param=off
      settings: xl_area=[0, 0, 0, 0, 0, 0, 0]
  Logical4 : xbsIndex_r3/Logical  logical_function=AND  inputs=2  precision=Full  arith_type=Unsigned  n_bits=8  bin_pt=2  align_bp=on  latency=0  explicit_period=on  period=1  en=off  dbl_ovrd=off  show_param=off
      settings: xl_area=[0, 0, 0, 0, 0, 0, 0]
  Logical9 : xbsIndex_r3/Logical  logical_function=AND  inputs=2  precision=Full  arith_type=Unsigned  n_bits=8  bin_pt=2  align_bp=on  latency=0  explicit_period=off  period=1  en=off  dbl_ovrd=off  show_param=off
      settings: xl_area=[0, 0, 0, 0, 0, 0, 0]
  Relational : xbsIndex_r3/Relational  mode=a=b  latency=0  explicit_period=off  period=1  en=off  dbl_ovrd=off  show_param=off
      settings: xl_area=[0, 0, 0, 0, 0, 0, 0]
  Slice1 : xbsIndex_r3/Slice  mode=Lower Bit Location + Width  nbits=13  bit1=0  base1=MSB of Input  bit0=0  base0=LSB of Input  boolean_output=off  explicit_period=off  period=1  dbl_ovrd=off
  Slice11 : xbsIndex_r3/Slice  mode=Lower Bit Location + Width  nbits=18  bit1=0  base1=MSB of Input  bit0=0  base0=LSB of Input  boolean_output=off  explicit_period=off  period=1  dbl_ovrd=off
  Slice12 : xbsIndex_r3/Slice  mode=Lower Bit Location + Width  nbits=16  bit1=0  base1=MSB of Input  bit0=0  base0=LSB of Input  boolean_output=off  explicit_period=off  period=1  dbl_ovrd=off
  Slice2 : xbsIndex_r3/Slice  mode=Lower Bit Location + Width  nbits=4  bit1=0  base1=MSB of Input  bit0=0  base0=LSB of Input  boolean_output=off  explicit_period=off  period=1  dbl_ovrd=off
  Slice3 : xbsIndex_r3/Slice  mode=Lower Bit Location + Width  nbits=16  bit1=0  base1=MSB of Input  bit0=0  base0=LSB of Input  boolean_output=off  explicit_period=off  period=1  dbl_ovrd=off
  Slice4 : xbsIndex_r3/Slice  mode=Two Bit Locations  nbits=11  bit1=chan_bits  base1=LSB of Input  bit0=xeng_bits  base0=LSB of Input  boolean_output=off  explicit_period=off  period=1  dbl_ovrd=off
  Slice5 : xbsIndex_r3/Slice  mode=Two Bit Locations  nbits=11  bit1=chan_bits  base1=LSB of Input  bit0=xeng_bits  base0=LSB of Input  boolean_output=off  explicit_period=off  period=1  dbl_ovrd=off
  Slice6 : xbsIndex_r3/Slice  mode=Lower Bit Location + Width  nbits=27  bit1=0  base1=MSB of Input  bit0=0  base0=LSB of Input  boolean_output=off  explicit_period=off  period=1  dbl_ovrd=off
  Slice7 : xbsIndex_r3/Slice  mode=Lower Bit Location + Width  nbits=13  bit1=0  base1=MSB of Input  bit0=0  base0=LSB of Input  boolean_output=off  explicit_period=off  period=1  dbl_ovrd=off
  Slice8 : xbsIndex_r3/Slice  mode=Lower Bit Location + Width  nbits=3  bit1=0  base1=MSB of Input  bit0=0  base0=LSB of Input  boolean_output=off  explicit_period=off  period=1  dbl_ovrd=off
  Slice9 : xbsIndex_r3/Slice  mode=Lower Bit Location + Width  nbits=11  bit1=0  base1=MSB of Input  bit0=0  base0=LSB of Input  boolean_output=off  explicit_period=off  period=1  dbl_ovrd=off
  Terminator1 : Terminator
  deflagger : Subsystem
  input_control : Subsystem
  output_control : Subsystem
  snap_rd : Subsystem  mask{nsamples=11}
      mask prompts: nsamples "Number of Samples (2^?)"
  snap_wr : Subsystem  mask{nsamples=12}
      mask prompts: nsamples "Number of Samples (2^?)"
  trig_freq : xps_library/software register  Tag=xps:sw_reg  io_dir=From Processor  arith_type=Unsigned  bitwidth=32  bin_pt=0  sample_period=1  gw_name=b_2x_8a_r310a_reord0_trig_freq_user_data_out
  dout : Outport
  valid : Outport  Port=2
  flag_out : Outport  Port=3
  rcvd : Outport  Port=4
  sync_out : Outport  Port=5
  max_mcnt : Outport  Port=6
  wires:
  input_control/4(we) -> Delay25/1
  input_control/2(wr_addr) -> Delay24/1
  output_control/2(rd_en) -> Dual Port RAM/3, Delay17/1, Delay18/1, Delay21/1
  output_control/3(rd_addr) -> Dual Port RAM/1, Delay16/1
  Constant/1 -> Dual Port RAM/2
  deflagger/3(rcvd) -> Convert5/1, rcvd/1, Inverter1/1
  deflagger/2(flag) -> flag_out/1, Convert4/1
  deflagger/1(dout) -> dout/1, Slice12/1
  Delay21/1 -> Convert3/1, valid/1, Logical9/1
  valid_in/1 -> input_control/1(valid), Delay11/1
  eof/1 -> input_control/2(eof), Delay15/1
  ant/1 -> input_control/4(ant), Delay13/1
  mcnt/1 -> input_control/3(mcnt), Delay14/1, Delay10/1
  Delay20/1 -> sync_out/1, Convert1/1
  Dual Port RAM/2 -> Terminator1/1
  Dual Port RAM/1 -> deflagger/1(din)
  output_control/1(gen_sync) -> Delay19/1, Delay20/1
  input_control/3(wr_data) -> Delay23/1
  din/1 -> input_control/6(data_in), Delay12/1
  flag/1 -> input_control/5(flag_in)
  input_control/1(maxcnt) -> output_control/1(maxcnt), Concat/1
  Concat/1 -> max_mcnt/1, Delay1/1
  Constant2/1 -> Concat/2
  Concat7/1 -> Delay2/1
  Delay4/1 -> snap_wr/2(we)
  Delay5/1 -> snap_wr/3(trig)
  Delay2/1 -> snap_wr/1(data_in)
  Slice9/1 -> Concat7/1
  Slice11/1 -> Concat7/2
  Convert2/1 -> Concat7/3
  Convert7/1 -> Concat7/4
  Slice1/1 -> Concat7/5
  Slice2/1 -> Concat7/6
  Slice3/1 -> Concat7/7
  Constant3/1 -> trig_freq/1
  Slice4/1 -> Relational/1
  trig_freq/1 -> Delay22/1
  Relational/1 -> Logical4/2
  Slice5/1 -> Relational/2
  Logical4/1 -> Delay5/1
  Concat1/1 -> Delay6/1
  Delay7/1 -> snap_rd/2(we)
  Delay8/1 -> snap_rd/3(trig)
  Delay6/1 -> snap_rd/1(data_in)
  Slice12/1 -> Concat1/3
  Slice7/1 -> Concat1/4
  Convert1/1 -> Concat1/5
  Convert3/1 -> Concat1/6
  Convert4/1 -> Concat1/7
  Convert5/1 -> Concat1/8
  Convert6/1 -> Concat1/9
  Slice6/1 -> Concat1/1
  Delay9/1 -> snap_rd/4(stop)
  output_control/4(current_rd_window) -> Delay3/1
  Slice8/1 -> Concat1/2
  Delay12/1 -> Delay29/1
  Delay13/1 -> Delay28/1
  Delay14/1 -> Delay27/1
  Delay15/1 -> Delay26/1
  Delay1/1 -> Slice6/1
  Delay3/1 -> Slice8/1
  Delay16/1 -> Slice7/1
  Delay17/1 -> Convert6/1
  Delay18/1 -> Delay7/1
  Delay19/1 -> Delay8/1
  Logical9/1 -> Delay9/1
  Inverter1/1 -> Logical9/2
  Delay11/1 -> Logical4/1, Delay4/1
  Delay10/1 -> Slice4/1
  Delay22/1 -> Slice5/1
  Delay24/1 -> Dual Port RAM/4, Slice9/1
  Delay23/1 -> Dual Port RAM/5, Slice11/1
  Delay25/1 -> Dual Port RAM/6, Convert2/1
  Delay26/1 -> Convert7/1
  Delay27/1 -> Slice1/1
  Delay28/1 -> Slice2/1
  Delay29/1 -> Slice3/1

== system test_pkt_reorder/descramble_orig/deflagger ==
  din : Inport  Port=1  LatchInput=off
  Slice1 : xbsIndex_r3/Slice  mode=Lower Bit Location + Width  nbits=16  bit1=0  base1=MSB of Input  bit0=0  base0=LSB of Input  boolean_output=off  explicit_period=on  period=1  dbl_ovrd=off
  Slice2 : xbsIndex_r3/Slice  mode=Upper Bit Location + Width  nbits=1  bit1=-1  base1=MSB of Input  bit0=0  base0=LSB of Input  boolean_output=off  explicit_period=on  period=1  dbl_ovrd=off
  Slice3 : xbsIndex_r3/Slice  mode=Upper Bit Location + Width  nbits=1  bit1=0  base1=MSB of Input  bit0=0  base0=LSB of Input  boolean_output=on  explicit_period=on  period=1  dbl_ovrd=off
  dout : Outport
  flag : Outport  Port=2
  rcvd : Outport  Port=3
  wires:
  Slice1/1 -> dout/1
  Slice3/1 -> rcvd/1
  Slice2/1 -> flag/1
  din/1 -> Slice3/1, Slice2/1, Slice1/1

== system test_pkt_reorder/descramble_orig/flagger ==
  flag : Inport  Port=1  LatchInput=off
  din : Inport  Port=2  LatchInput=off
  Concat : xbsIndex_r3/Concat  num_inputs=12  explicit_period=off  period=1  dbl_ovrd=off
  Constant{1..4} (4 alike) : xbsIndex_r3/Constant  const=1  equ=P=C  arith_type=Unsigned  n_bits=1  bin_pt=0  opselect=C  inp2=PCIN>>17  opr=+  inp1=P  carry=CIN  iostate=0  explicit_period=on  period=1  dbl_ovrd=off
  Slice1 : xbsIndex_r3/Slice  mode=Lower Bit Location + Width  nbits=16  bit1=0  base1=MSB of Input  bit0=0  base0=LSB of Input  boolean_output=off  explicit_period=off  period=1  dbl_ovrd=off
  Slice2 : xbsIndex_r3/Slice  mode=Lower Bit Location + Width  nbits=16  bit1=0  base1=MSB of Input  bit0=16  base0=LSB of Input  boolean_output=off  explicit_period=off  period=1  dbl_ovrd=off
  Slice3 : xbsIndex_r3/Slice  mode=Lower Bit Location + Width  nbits=16  bit1=0  base1=MSB of Input  bit0=32  base0=LSB of Input  boolean_output=off  explicit_period=off  period=1  dbl_ovrd=off
  Slice4 : xbsIndex_r3/Slice  mode=Lower Bit Location + Width  nbits=16  bit1=0  base1=MSB of Input  bit0=48  base0=LSB of Input  boolean_output=off  explicit_period=off  period=1  dbl_ovrd=off
  dout : Outport
  wires:
  Concat/1 -> dout/1
  din/1 -> Slice4/1, Slice3/1, Slice2/1, Slice1/1
  flag/1 -> Concat/11, Concat/8, Concat/5, Concat/2
  Slice4/1 -> Concat/12
  Slice3/1 -> Concat/9
  Slice2/1 -> Concat/6
  Slice1/1 -> Concat/3
  Constant1/1 -> Concat/10
  Constant2/1 -> Concat/7
  Constant3/1 -> Concat/4
  Constant4/1 -> Concat/1
